simulink model "ass6_5"  (R2023a)
settings: Solver=VariableStepAuto  StartTime=0.0  StopTime=10.0  RelTol=1e-3
settings Model: Creator=Taniya Baral  LastModifiedBy=Taniya Baral

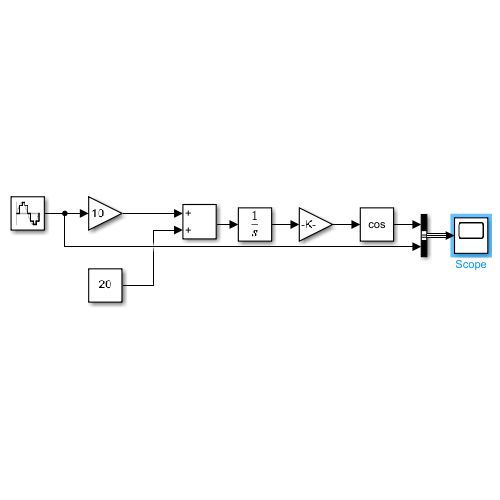
[thumbnail: Simulink's stored preview of the top-level diagram]
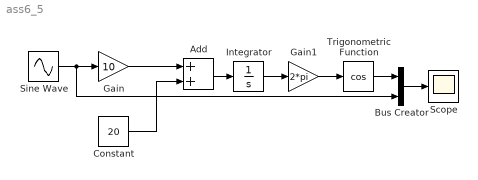
== system ass6_5 ==
  Add : Sum
  Bus Creator : BusCreator  Inputs=2
  Constant : Constant  Value=20
  Gain : Gain  Gain=10
  Gain1 : Gain  Gain=2*pi
  Integrator : Integrator
  Scope : Scope
  Sine Wave : Sin  Frequency=2*pi  SampleTime=180
  Trigonometric Function : Trigonometry  Operator=cos
  wires:
  Add/1 -> Integrator/1
  Integrator/1 -> Gain1/1
  Gain1/1 -> Trigonometric Function/1
  Sine Wave/1 -> Bus Creator/2, Gain/1
  Gain/1 -> Add/1
  Constant/1 -> Add/2
  Trigonometric Function/1 -> Bus Creator/1
  Bus Creator/1 -> Scope/1
